simulink model "second_cl_2"  (R2021a)
settings: Solver=VariableStepAuto  StartTime=0.0  StopTime=20  RelTol=1e-3
values from neighbouring files (symbols this model uses):
  K = lqr_controller(sys)    [ex3main.m]
  params = get_params()    [ex3main.m]
  sys = get_system(params)    [ex3main.m]
  Ts = 1/200    (= 0.005)    [ex3main.m]
  wc = 2*f*pi    (= 12.5663706144)    [ex3main.m]
  x_d = desired_state(theta_d, params)    [ex3main.m]
undefined symbols (not defined in the file or in its folder): dist
libraries: simulink x2
settings Model: Creator=martijndebeuf  LastModifiedBy=Gebruiker
settings SolverCC: AlgebraicLoopSolver=TrustRegion
settings DebuggingCC: SFMachineParentedDataDiag=warning

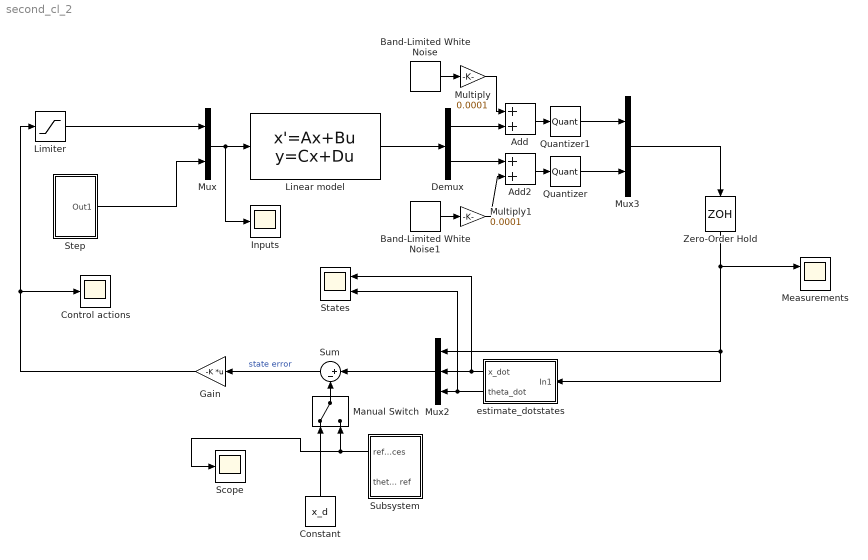
== system second_cl_2 ==
  Add : Sum
  Add2 : Sum
  Band-Limited White Noise : simulink/Sources/Band-Limited White Noise  Cov=[0.1]  Ts=Ts  seed=[23341]
  Band-Limited White Noise1 : simulink/Sources/Band-Limited White Noise  Cov=[0.1]  Ts=Ts  seed=[23342]
  Constant : Constant  Value=x_d  SampleTime=Ts
  Control actions : Scope
  Demux : Demux  Outputs=2
  Gain : Gain  Gain=-K  Multiplication=Matrix(K*u) (u vector)
  Inputs : Scope
  Limiter : Saturate  UpperLimit=5  LowerLimit=-5
  Linear model : StateSpace  A=sys.A  B=[sys.B,dist]  C=sys.C  D=[sys.D,zeros(2,1)]  InitialCondition=initial_conditions'
  Manual Switch : ManualSwitch
  Measurements : Scope  NumInputPorts=2
  Multiply : Gain  Gain=0.0001
  Multiply1 : Gain  Gain=0.0001
  Mux : Mux  Inputs=2
  Mux2 : Mux  Inputs=3
  Mux3 : Mux  Inputs=2
  Quantizer : Quantizer  QuantizationInterval=resolutiontheta
  Quantizer1 : Quantizer  QuantizationInterval=resolutionx
  Scope : Scope
  States : Scope  NumInputPorts=2
  Step : Subsystem
  Subsystem : Subsystem
  Sum : Sum  Inputs=|+-
  Zero-Order Hold : ZeroOrderHold  SampleTime=Ts
  estimate_dotstates : Subsystem
  wires:
  Mux/1 -> Inputs/1, Linear model/1
  Add2/1 -> Quantizer/1
  Limiter/1 -> Mux/1
  Band-Limited White Noise/1 -> Multiply/1
  Gain/1 -> Limiter/1, Control actions/1
  Multiply/1 -> Add/1
  Band-Limited White Noise1/1 -> Multiply1/1
  Demux/1 -> Add/2
  Linear model/1 -> Demux/1
  Demux/2 -> Add2/1
  Quantizer1/1 -> Mux3/1
  Sum/1 -> Gain/1  "state error"
  Quantizer/1 -> Mux3/2
  Add/1 -> Quantizer1/1
  Multiply1/1 -> Add2/2
  Mux3/1 -> Zero-Order Hold/1
  Zero-Order Hold/1 -> estimate_dotstates/1(In1), Mux2/1, Measurements/1
  Mux2/1 -> Sum/1
  Step/1(Out1) -> Mux/2
  Subsystem/1(references) -> Manual Switch/2, Scope/1
  estimate_dotstates/1(x_dot) -> Mux2/2, States/1
  estimate_dotstates/2(theta_dot) -> Mux2/3, States/2
  Manual Switch/1 -> Sum/2
  Constant/1 -> Manual Switch/1

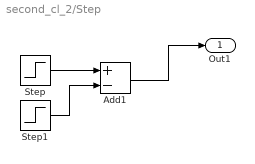
== system second_cl_2/Step ==
  Add1 : Sum  Inputs=+-
  Step : Step  Time=3  SampleTime=Ts
  Step1 : Step  Time=3.1  SampleTime=Ts
  Out1 : Outport
  wires:
  Step/1 -> Add1/1
  Add1/1 -> Out1/1
  Step1/1 -> Add1/2

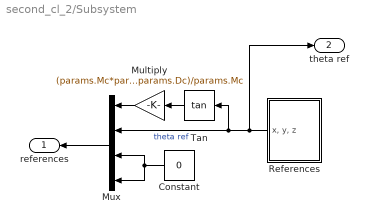
== system second_cl_2/Subsystem ==
  Constant : Constant  Value=0
  Multiply : Gain  Gain=(params.Mc*params.Dt+params.Msw*params.Dc)/params.Mc
  Mux : Mux
  References : Subsystem
  Tan : Trigonometry  Operator=tan
  references : Outport
  theta ref : Outport  Port=2
  wires:
  Mux/1 -> references/1
  Tan/1 -> Multiply/1
  Multiply/1 -> Mux/1
  References/1("x, y, z") -> theta ref/1, Tan/1, Mux/2  "theta ref"
  Constant/1 -> Mux/4, Mux/3

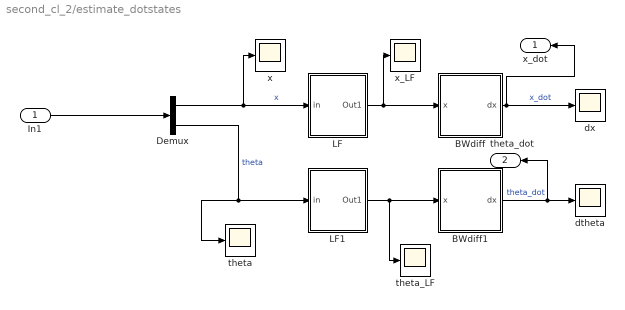
== system second_cl_2/estimate_dotstates ==
  In1 : Inport
  BWdiff : Subsystem
  BWdiff1 : Subsystem
  Demux : Demux  Outputs=2
  LF : Subsystem
  LF1 : Subsystem
  dtheta : Scope
  dx : Scope
  theta : Scope
  theta_LF : Scope
  x : Scope
  x_LF : Scope
  x_dot : Outport
  theta_dot : Outport  Port=2
  wires:
  LF1/1(Out1) -> theta_LF/1, BWdiff1/1(x)
  Demux/2 -> LF1/1(in), theta/1  "theta"
  BWdiff1/1(dx) -> theta_dot/1, dtheta/1  "theta_dot"
  LF/1(Out1) -> x_LF/1, BWdiff/1(x)
  BWdiff/1(dx) -> x_dot/1, dx/1  "x_dot"
  Demux/1 -> LF/1(in), x/1  "x"
  In1/1 -> Demux/1

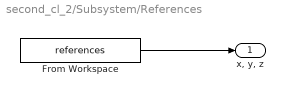
== system second_cl_2/Subsystem/References ==
  From Workspace : FromWorkspace  VariableName=references  SampleTime=Ts  Interpolate=off  OutputAfterFinalValue=Holding final value
  "x, y, z" : Outport
  wires:
  From Workspace/1 -> "x, y, z"/1

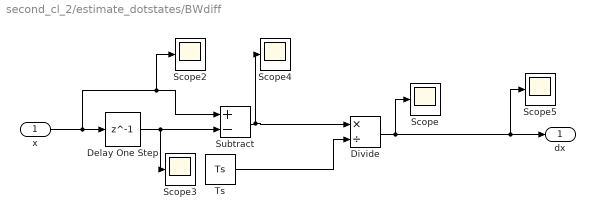
== system second_cl_2/estimate_dotstates/BWdiff ==
  x : Inport
  Delay One Step : Delay  DelayLength=1
  Divide : Product  Inputs=*/
  Scope{,2..5} (5 alike) : Scope
  Subtract : Sum  Inputs=+-
  Ts : Constant  Value=Ts
  dx : Outport
  wires:
  Delay One Step/1 -> Scope3/1, Subtract/2
  Ts/1 -> Divide/2
  x/1 -> Delay One Step/1, Scope2/1, Subtract/1
  Subtract/1 -> Divide/1, Scope4/1
  Divide/1 -> Scope5/1, dx/1, Scope/1

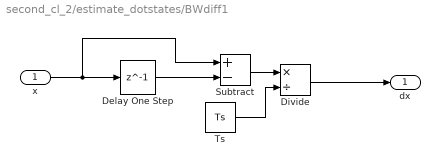
== system second_cl_2/estimate_dotstates/BWdiff1 ==
  x : Inport
  Delay One Step : Delay  DelayLength=1
  Divide : Product  Inputs=*/
  Subtract : Sum  Inputs=+-
  Ts : Constant  Value=Ts
  dx : Outport
  wires:
  Ts/1 -> Divide/2
  Subtract/1 -> Divide/1
  x/1 -> Delay One Step/1, Subtract/1
  Divide/1 -> dx/1
  Delay One Step/1 -> Subtract/2

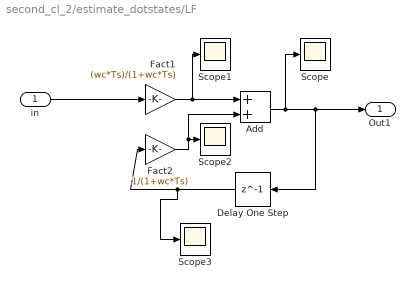
== system second_cl_2/estimate_dotstates/LF ==
  in : Inport
  Add : Sum
  Delay One Step : Delay  DelayLength=1
  Fact1 : Gain  Gain=(wc*Ts)/(1+wc*Ts)
  Fact2 : Gain  Gain=1/(1+wc*Ts)
  Scope{,1..3} (4 alike) : Scope
  Out1 : Outport
  wires:
  Fact2/1 -> Add/2, Scope2/1
  Fact1/1 -> Scope1/1, Add/1
  in/1 -> Fact1/1
  Add/1 -> Scope/1, Delay One Step/1, Out1/1
  Delay One Step/1 -> Scope3/1, Fact2/1

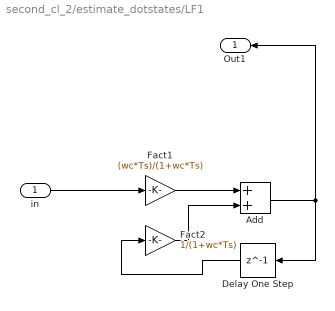
== system second_cl_2/estimate_dotstates/LF1 ==
  in : Inport
  Add : Sum
  Delay One Step : Delay  DelayLength=1
  Fact1 : Gain  Gain=(wc*Ts)/(1+wc*Ts)
  Fact2 : Gain  Gain=1/(1+wc*Ts)
  Out1 : Outport
  wires:
  Add/1 -> Delay One Step/1, Out1/1
  Fact2/1 -> Add/2
  Fact1/1 -> Add/1
  in/1 -> Fact1/1
  Delay One Step/1 -> Fact2/1
